simulink model "fixpt_autoscale_bk"  (R2015b)
settings: Solver=FixedStepDiscrete  SolverMode=SingleTasking  StartTime=0.0  StopTime=10  RelTol=1e-3
PreLoadFcn:
  | [num,den] = butter(1,0.3);
libraries: simulink x1
settings Model: Creator=y_yama  LastModifiedBy=amatsumo
settings DataIOCC: SaveFormat=Array  SignalLoggingSaveFormat=ModelDataLogs  SaveOutput=off  SignalLogging=off  SaveTime=off
settings OptimizationCC: BlockReduction=off  ConditionallyExecuteInputs=off  DefaultParameterBehavior=Inlined  InlineInvariantSignals=on  ExpressionDepthLimit=2147483647  ZeroExternalMemoryAtStartup=off  ZeroInternalMemoryAtStartup=off  InitFltsAndDblsToZero=on  NoFixptDivByZeroProtection=on  EfficientFloat2IntCast=on  OptimizeModelRefInitCode=on  LifeSpan=1
settings DebuggingCC: AlgebraicLoopMsg=error  UnderspecifiedInitializationDetection=Classic  MergeDetectMultiDrivingBlocksExec=none  SolverPrmCheckMsg=warning  InheritedTsInSrcMsg=none  SingleTaskRateTransMsg=error  ParameterPrecisionLossMsg=none  FcnCallInpInsideContextMsg=UseLocalSettings  StateNameClashWarn=warning
settings HardwareCC: ProdBitPerPointer=32  ProdLargestAtomicFloat=None  ProdIntDivRoundTo=Undefined  ProdEndianess=Unspecified  ProdWordSize=32  ProdHWDeviceType=ASIC/FPGA->ASIC/FPGA  TargetBitPerPointer=64  TargetLongLongMode=on  TargetIntDivRoundTo=Zero  TargetEndianess=LittleEndian  TargetWordSize=64  TargetHWDeviceType=MATLAB Host  ProdEqTarget=off
settings RTWCC: SystemTargetFile=ert.tlc  GenCodeOnly=on  TemplateMakefile=ert_default_tmf  Description=Real-Time Workshop Embedded Coder (no auto configuration)  GenerateReport=on  IncludeHyperlinkInReport=on  LaunchReport=on
settings CodeAppCC: GenerateComments=off  IgnoreCustomStorageClasses=off  CustomSymbolStrGlobalVar=$N$M  CustomSymbolStrType=$N$R$M  SimulinkBlockComments=off  InternalIdentifier=Classic
settings ERTTargetCC: GenerateSampleERTMain=on  IncludeMdlTerminateFcn=off  SuppressErrorStatus=on  SupportAbsoluteTime=off  SupportNonFinite=off  SupportComplex=off  PurelyIntegerCode=on  InlinedParameterPlacement=NonHierarchical  ERTCustomFileTemplate=example_file_process.tlc
settings ConfigComp: CovModelRefEnable=Off  CovSFcnEnable=off

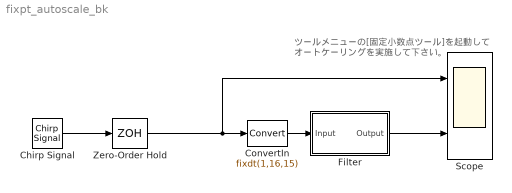
== system fixpt_autoscale_bk ==
  note: ツールメニューの[固定小数点ツール]を起動して
      | オートケーリングを実施して下さい。
  Chirp Signal : simulink/Sources/Chirp Signal  f1=10  T=10  f2=500
  ConvertIn : DataTypeConversion  OutDataTypeStr=fixdt(1,16,15)  RndMeth=Nearest  SaturateOnIntegerOverflow=on
  Filter : Subsystem  Tag=FilterWizardSubSystem  TreatAsAtomicUnit=on
  Scope : Scope  NumInputPorts=2
  Zero-Order Hold : ZeroOrderHold  SampleTime=1/1000
  wires:
  Filter/1(Output) -> Scope/2
  Chirp Signal/1 -> Zero-Order Hold/1
  ConvertIn/1 -> Filter/1(Input)
  Zero-Order Hold/1 -> Scope/1, ConvertIn/1

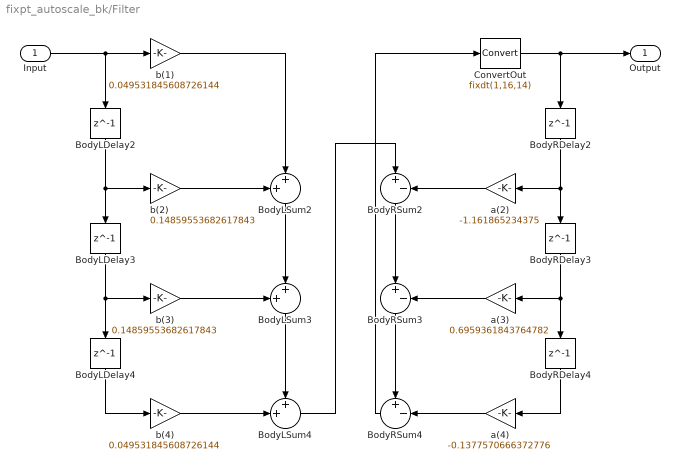
== system fixpt_autoscale_bk/Filter ==
  Input : Inport
  BodyLDelay2 : Delay  DelayLength=1  InitialCondition=0
  BodyLDelay3 : Delay  DelayLength=1  InitialCondition=0
  BodyLDelay4 : Delay  DelayLength=1  InitialCondition=0
  BodyLSum2 : Sum  Inputs=++|  AccumDataTypeStr=fixdt(1,40,32)  OutDataTypeStr=fixdt(1,40,32)  RndMeth=Convergent
  BodyLSum3 : Sum  Inputs=++|  AccumDataTypeStr=fixdt(1,40,32)  OutDataTypeStr=fixdt(1,40,32)  RndMeth=Convergent
  BodyLSum4 : Sum  Inputs=++|  AccumDataTypeStr=fixdt(1,40,32)  OutDataTypeStr=fixdt(1,40,32)  RndMeth=Convergent
  BodyRDelay2 : Delay  DelayLength=1  InitialCondition=0
  BodyRDelay3 : Delay  DelayLength=1  InitialCondition=0
  BodyRDelay4 : Delay  DelayLength=1  InitialCondition=0
  BodyRSum2 : Sum  Inputs=|+-  AccumDataTypeStr=fixdt(1,40,32)  OutDataTypeStr=fixdt(1,40,32)  RndMeth=Convergent
  BodyRSum3 : Sum  Inputs=|+-  AccumDataTypeStr=fixdt(1,40,32)  OutDataTypeStr=fixdt(1,40,32)  RndMeth=Convergent
  BodyRSum4 : Sum  Inputs=+-|  AccumDataTypeStr=fixdt(1,40,32)  OutDataTypeStr=fixdt(1,40,32)  RndMeth=Convergent
  ConvertOut : DataTypeConversion  OutDataTypeStr=fixdt(1,16,14)  RndMeth=Convergent
  a(2) : Gain  Gain=-1.161865234375  ParamDataTypeStr=fixdt(1,16,14)  OutDataTypeStr=fixdt(1,32,32)  RndMeth=Convergent
  a(3) : Gain  Gain=0.6959361843764782  ParamDataTypeStr=fixdt(1,16,14)  OutDataTypeStr=fixdt(1,32,32)  RndMeth=Convergent
  a(4) : Gain  Gain=-0.1377570666372776  ParamDataTypeStr=fixdt(1,16,14)  OutDataTypeStr=fixdt(1,32,32)  RndMeth=Convergent
  b(1) : Gain  Gain=0.049531845608726144  ParamDataTypeStr=fixdt(1,16,17)  OutDataTypeStr=fixdt(1,32,32)  RndMeth=Convergent
  b(2) : Gain  Gain=0.14859553682617843  ParamDataTypeStr=fixdt(1,16,17)  OutDataTypeStr=fixdt(1,32,32)  RndMeth=Convergent
  b(3) : Gain  Gain=0.14859553682617843  ParamDataTypeStr=fixdt(1,16,17)  OutDataTypeStr=fixdt(1,32,32)  RndMeth=Convergent
  b(4) : Gain  Gain=0.049531845608726144  ParamDataTypeStr=fixdt(1,16,17)  OutDataTypeStr=fixdt(1,32,32)  RndMeth=Convergent
  Output : Outport
  wires:
  b(1)/1 -> BodyLSum2/2
  ConvertOut/1 -> Output/1, BodyRDelay2/1
  Input/1 -> b(1)/1, BodyLDelay2/1
  BodyLDelay2/1 -> BodyLDelay3/1, b(2)/1
  b(2)/1 -> BodyLSum2/1
  BodyLSum2/1 -> BodyLSum3/2
  BodyRSum2/1 -> BodyRSum3/1
  a(2)/1 -> BodyRSum2/2
  BodyRDelay2/1 -> a(2)/1, BodyRDelay3/1
  BodyLDelay3/1 -> BodyLDelay4/1, b(3)/1
  b(3)/1 -> BodyLSum3/1
  BodyLSum3/1 -> BodyLSum4/1
  BodyRSum3/1 -> BodyRSum4/1
  a(3)/1 -> BodyRSum3/2
  BodyRDelay3/1 -> a(3)/1, BodyRDelay4/1
  BodyLDelay4/1 -> b(4)/1
  b(4)/1 -> BodyLSum4/2
  BodyLSum4/1 -> BodyRSum2/1
  BodyRSum4/1 -> ConvertOut/1
  a(4)/1 -> BodyRSum4/2
  BodyRDelay4/1 -> a(4)/1
